simulink model "SimETC"  (R2025b)
settings: Solver=FixedStepAuto  StartTime=0.0  StopTime=50  FixedStep=Ts  RelTol=1e-3
values from neighbouring files (symbols this model uses):
  hiddenLayerSizeCtrl = 20    [Init.m]
  hiddenLayerSizeObsv = 5    [Init.m]
  n = 2    [Init.m]
  p = 1    [Init.m]
  Ts = 1e-3    (= 0.001)    [Init.m]
  u_max = 5    [Init.m]
  u_min = - 5    (= -5)    [Init.m]
  Vctrl0 = 0.1 * randn(hiddenLayerSizeCtrl, inputLayerSizeCtrl)    [Init.m]
  Vobsv0 = 0.1 * randn(hiddenLayerSizeObsv, inputLayerSizeObsv)    [Init.m]
  Wctrl0 = 0.1 * randn(outputLayerSizeCtrl, hiddenLayerSizeCtrl)    [Init.m]
  Wobsv0 = 0.1 * randn(outputLayerSizeObsv, hiddenLayerSizeObsv)    [Init.m]
  x0 = [0.5; 0]    [Init.m]
  x_hat0 = [0.9; 0]    [Init.m]
settings Model: Creator=Asus  LastModifiedBy=Asus

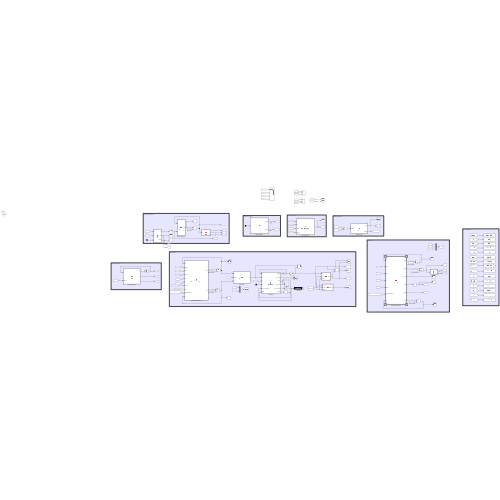
[thumbnail: Simulink's stored preview of the top-level diagram]
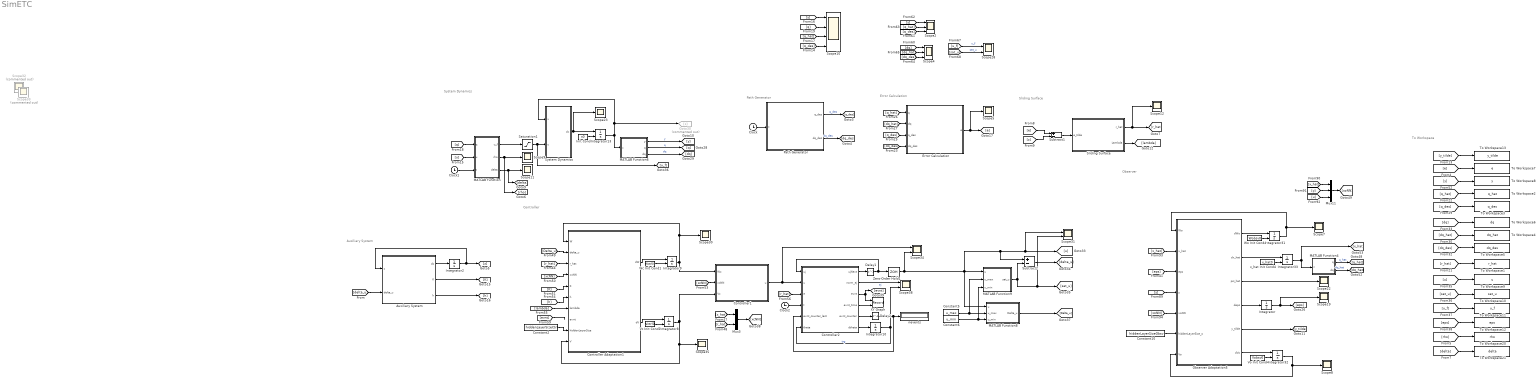
== system SimETC ==
  note: Path Generator
  note: Auxiliary System
  note: Sliding Surface
  note: Error Calculation
  note: Observer
  note: System Dynamics
  note: To Workspace
  note: Controller
  Auxiliary System : MATLAB Function  TreatAsAtomicUnit=on
  Clock : Clock
  Clock1 : Clock
  Clock2 : Clock
  Constant10 : Constant  Value=hiddenLayerSizeObsv
  Constant2 : Constant  Value=hiddenLayerSizeCtrl
  Constant5 : Constant  Value=u_max
  Constant6 : Constant  Value=u_min
  Controller Adaptation1 : MATLAB Function  TreatAsAtomicUnit=on
  Controller1 : MATLAB Function  TreatAsAtomicUnit=on
  Controller2 : MATLAB Function  TreatAsAtomicUnit=on
  Delay1 : Delay  DelayLength=1  InitialCondition=0  SampleTime=Ts
  Delay2 : Delay  DelayLength=1  InitialCondition=0  SampleTime=Ts
  Error Calculation : MATLAB Function  TreatAsAtomicUnit=on
  Goto30 : Goto  Commented=on  GotoTag=x
  Init Cond : Constant  Value=x0
  Integrator : Integrator  InitialCondition=5 * ones(p, 1)
  Integrator10 : Integrator  InitialCondition=1
  Integrator{13,31..33} (4 alike) : Integrator  InitialConditionSource=external  InitialCondition=[0.5; 0.5]
  Integrator2 : Integrator  InitialCondition=zeros(n, 1)
  Integrator8 : Integrator  InitialConditionSource=external
  Integrator9 : Integrator  InitialConditionSource=external
  MATLAB Function : MATLAB Function  TreatAsAtomicUnit=on
  MATLAB Function4 : MATLAB Function  TreatAsAtomicUnit=on
  MATLAB Function6 : MATLAB Function  TreatAsAtomicUnit=on
  MATLAB Function8 : MATLAB Function  TreatAsAtomicUnit=on
  MATLAB Function9 : MATLAB Function  TreatAsAtomicUnit=on
  Mux11 : Mux  Inputs=3
  Mux3 : Mux  Inputs=2
  Observer Adaptation5 : MATLAB Function  TreatAsAtomicUnit=on
  Path Generator : MATLAB Function  TreatAsAtomicUnit=on
  Saturation1 : Saturate  UpperLimit=u_max  LowerLimit=u_min
  Scope10 : Scope  NumInputPorts=4
      settings: ActiveDisplayYMinimum=-1.6367696892605232  ActiveDisplayYMaximum=1.5189809741527545  DataLoggingVariableName=ScopeData11
  Scope{5,7..9,11..12,19,22..23,30,35} (11 alike) : Scope
      Scope11 settings: ActiveDisplayYMinimum=-0.44130868539267287  ActiveDisplayYMaximum=0.66139690029774989  DataLoggingVariableName=ScopeData6
      Scope12 settings: ActiveDisplayYMinimum=-17.664742140770244  ActiveDisplayYMaximum=31.96274912675225  DataLoggingVariableName=ScopeData7
      Scope19 settings: ActiveDisplayYMinimum=1.4821345739344274  ActiveDisplayYMaximum=36.660788834590164  DataLoggingVariableName=ScopeData15
      Scope22 settings: ActiveDisplayYMinimum=-0.17253514431660325  ActiveDisplayYMaximum=0.24898535652907006  DataLoggingVariableName=ScopeData18
      Scope23 settings: ActiveDisplayYMinimum=-17.129349977314451  ActiveDisplayYMaximum=21.988712096819278  DataLoggingVariableName=ScopeData19
      Scope30 settings: ActiveDisplayYMinimum=-1.927386800082266  ActiveDisplayYMaximum=2.0755368522631517  DataLoggingVariableName=ScopeData29
      Scope35 settings: ActiveDisplayYMinimum=-1  ActiveDisplayYMaximum=1  DataLoggingVariableName=ScopeData34
      Scope5 settings: ActiveDisplayYMinimum=-0.81519678925710282  ActiveDisplayYMaximum=0.81279964325078913
      Scope7 settings: ActiveDisplayYMinimum=-0.11116662287651718  ActiveDisplayYMaximum=0.13560443561010163  DataLoggingVariableName=ScopeData9
      Scope8 settings: ActiveDisplayYMinimum=-0.37596192997099781  ActiveDisplayYMaximum=0.43937320774408428  DataLoggingVariableName=ScopeData10
      Scope9 settings: ActiveDisplayYMinimum=0.66977640233126912  ActiveDisplayYMaximum=1.0366915108520809  DataLoggingVariableName=ScopeData5
  Scope2 : Scope  NumInputPorts=3
      settings: ActiveDisplayYMinimum=-0.95485365659347476  ActiveDisplayYMaximum=1.1060948507326083
  Scope{28,31,34,38} (4 alike) : Scope  NumInputPorts=2
      Scope28 settings: ActiveDisplayYMinimum=-6.25  ActiveDisplayYMaximum=6.25  DataLoggingVariableName=ScopeData24
      Scope31 settings: ActiveDisplayYMinimum=-16.631670131101757  ActiveDisplayYMaximum=15.404984351853386  DataLoggingVariableName=ScopeData30
      Scope34 settings: ActiveDisplayYMinimum=-1.1199808946106344  ActiveDisplayYMaximum=-0.23536958662686125  DataLoggingVariableName=ScopeData33
      Scope38 settings: ActiveDisplayYMinimum=-0.40772759021012284  ActiveDisplayYMaximum=3.6695544974688574  DataLoggingVariableName=ScopeData37
  Scope32 : Scope  Commented=on
      settings: ActiveDisplayYMinimum=-0.12499999999999997  ActiveDisplayYMaximum=1.125  DataLoggingVariableName=ScopeData31
  Scope33 : Scope  Commented=on
      settings: ActiveDisplayYMinimum=-0.12499999999999997  ActiveDisplayYMaximum=1.125  DataLoggingVariableName=ScopeData32
  Scope4 : Scope  NumInputPorts=3
      settings: ActiveDisplayYMinimum=-2.1086647102859288  ActiveDisplayYMaximum=2.2459506500821029  DataLoggingVariableName=ScopeData8
  Sliding Surface : MATLAB Function  TreatAsAtomicUnit=on
  Subtract1 : Sum  Inputs=+-
  Subtract2 : Sum  Inputs=+-
  System Dynamics : MATLAB Function  TreatAsAtomicUnit=on
  To Workspace1 : ToWorkspace  VariableName=r_hat  SaveFormat=Structure  SampleTime=-1
      settings: Save2DSignal=2-D array (concatenate along first dimension)
  To Workspace10 : ToWorkspace  VariableName=sat_u  SaveFormat=Structure  SampleTime=-1
      settings: Save2DSignal=2-D array (concatenate along first dimension)
  To Workspace11 : ToWorkspace  VariableName=u_f  SaveFormat=Structure  SampleTime=-1
      settings: Save2DSignal=2-D array (concatenate along first dimension)
  To Workspace12 : ToWorkspace  VariableName=eps  SaveFormat=Structure  SampleTime=-1
      settings: Save2DSignal=2-D array (concatenate along first dimension)
  To Workspace13 : ToWorkspace  VariableName=y_tilde  SaveFormat=Structure  SampleTime=-1
      settings: Save2DSignal=2-D array (concatenate along first dimension)
  To Workspace2 : ToWorkspace  VariableName=q_hat  SaveFormat=Structure  SampleTime=-1
      settings: Save2DSignal=2-D array (concatenate along first dimension)
  To Workspace20 : ToWorkspace  VariableName=rho  SaveFormat=Structure  SampleTime=-1
      settings: Save2DSignal=2-D array (concatenate along first dimension)
  To Workspace21 : ToWorkspace  VariableName=delta  SaveFormat=Structure  SampleTime=-1
      settings: Save2DSignal=2-D array (concatenate along first dimension)
  To Workspace3 : ToWorkspace  VariableName=q_des  SaveFormat=Structure  SampleTime=-1
      settings: Save2DSignal=2-D array (concatenate along first dimension)
  To Workspace4 : ToWorkspace  VariableName=dq_hat  SaveFormat=Structure  SampleTime=-1
      settings: Save2DSignal=2-D array (concatenate along first dimension)
  To Workspace5 : ToWorkspace  VariableName=dq_des  SaveFormat=Structure  SampleTime=-1
      settings: Save2DSignal=2-D array (concatenate along first dimension)
  To Workspace6 : ToWorkspace  VariableName=dq  SaveFormat=Structure  SampleTime=-1
      settings: Save2DSignal=2-D array (concatenate along first dimension)
  To Workspace7 : ToWorkspace  VariableName=e  SaveFormat=Structure  SampleTime=-1
      settings: Save2DSignal=2-D array (concatenate along first dimension)
  To Workspace8 : ToWorkspace  VariableName=y  SaveFormat=Structure  SampleTime=-1
      settings: Save2DSignal=2-D array (concatenate along first dimension)
  To Workspace9 : ToWorkspace  VariableName=u  SaveFormat=Structure  SampleTime=-1
      settings: Save2DSignal=2-D array (concatenate along first dimension)
  Vc Init Cond1 : Constant  Value=Vctrl0
  Vo Init Cond4 : Constant  Value=Vobsv0
  Wc Init Cond1 : Constant  Value=Wctrl0
  Wo Init Cond4 : Constant  Value=Wobsv0
  XY Graph : Record  NumPorts=2.0  FileSettingsInternal="{\"entries\":[{\"content\":{\"excelSettings\":{\"content\":{},\"type\":\"Streamout.ExcelSettings\"},\"parquetSettings\":{\"content\":{},\"type\":\"Streamout.ParquetSettings\"}},\"type\":\"Streamout.FileSettingStorage\",\"uuid\":\"\"}],\"packageUris\":[\"http:\\/\\/schema.mathworks.com\\/mf0\\/streamout_blocks\\/R2020a\"],\"version\":\"1.0\"}"  FrameSettings=[0, 0]  Layout=[1 1]  SignalsInternal="{\"entries\":[{\"content\":{\"signals\":[{\"content\":{\"blockPath\":[],\"dimensions\":[1],\"domain\":\"\",\"lineColor\":\"#a2142f\",\"plots\":[ 1 ],\"port\":1,\"sid\":[\"\"],\"signalID\":1,\"signalName\":\"Controller2:3\"},\"type\":\"RecordBlkView.Signal\",\"uuid\":\"\"},{\"content\":{\"blockPath\":[],\"dimensions\":[1],\"domain\":\"\",\"lineColor\":\"#139fff\",\"plots\":[ 1 ],\"port\":2,\"sid\":[\"\"],\"signalID\":2,\"signalName\":\"Controller2:4\"},\"type\":\"RecordBlkView.Signal\",\"uuid\":\"\"}]},\"type\":\"RecordBlkView.InputSignals\",\"uuid\":\"\"}],\"packageUris\":[\"http:\\/\\/schema.mathworks.com\\/mf0\\/streamout_blocks\\/R2020a\"],\"version\":\"1.0\"}"  VisualizationBindings="{\"xyplotplugin\":{\"info\":[{\"series\":[{\"bindingParametersList\":[{\"parameter\":\"X-Axis\",\"signalID\":1,\"signalName\":\"Controller2:3\"},{\"parameter\":\"Y-Axis\",\"signalID\":2,\"signalName\":\"Controller2:4\"}],\"seriesID\":0}],\"subplotID\":1}]}}"  CompatibilityTag=XY
  Zero-Order Hold1 : ZeroOrderHold  SampleTime=Ts
  nevents : Display
  x_hat Init Cond4 : Constant  Value=x_hat0
  wires:
  Clock/1 -> Path Generator/1(t)
  Auxiliary System/1(dz) -> Integrator2/1
  Integrator2/1 -> [z], Auxiliary System/1(z)
  Sliding Surface/1(r_hat) -> Scope12/1, [r_hat]
  Path Generator/2(dq_des) -> [dq_des]  "dq_des"
  Path Generator/1(q_des) -> [q_des]  "q_des"
  Sliding Surface/2(Lambda) -> [lambda]
  Error Calculation/1(e) -> Scope5/1, [e]
  [q_des] -> Error Calculation/3(q_des)
  [dq_des] -> Error Calculation/4(dq_des)
  [delta_u] -> Auxiliary System/2(delta_u)
  [dq_hat] -> Error Calculation/2(dq)
  Observer Adaptation5/2(dx_hat) -> Integrator33/1
  Observer Adaptation5/6(dVo) -> Integrator32/1
  Mux11/1 -> [xoNN]
  MATLAB Function4/2(dq) -> [dq_hat]  "dq_hat"
  [xoNN] -> Observer Adaptation5/5(xoNN)
  Integrator32/1 -> Observer Adaptation5/7(Vo), Scope8/1
  MATLAB Function4/1(q) -> [q_hat]  "q_hat"
  [u] -> Mux11/3
  [y] -> Observer Adaptation5/4(y)
  Wo Init Cond4/1 -> Integrator31/2
  Constant10/1 -> Observer Adaptation5/6(hiddenLayerSize_o)
  [x_hat] -> Observer Adaptation5/2(x_hat)
  Integrator31/1 -> Scope7/1, Observer Adaptation5/1(Wo)
  x_hat Init Cond4/1 -> Integrator33/2
  [x_hat] -> Mux11/1
  Vo Init Cond4/1 -> Integrator32/2
  [y] -> Mux11/2
  [q_hat] -> Error Calculation/1(q)
  MATLAB Function6/2(q) -> [q]  "q"
  Integrator13/1 -> System Dynamics/1(x), Goto30/1, MATLAB Function6/1(x)
  System Dynamics/1(dx) -> Scope23/1, Integrator13/1
  MATLAB Function6/3(dq) -> [dq]  "dq"
  Init Cond/1 -> Integrator13/2
  Observer Adaptation5/1(dWo) -> Integrator31/1
  Integrator33/1 -> MATLAB Function4/1(x), [x_hat]
  Observer Adaptation5/4(deps) -> Integrator/1
  Integrator/1 -> Scope19/1, [eps]
  [eps] -> Observer Adaptation5/3(eps)
  Observer Adaptation5/3(psi_hat) -> Scope22/1
  [e] -> Subtract1/1
  Subtract1/1 -> Sliding Surface/1(e_tilde)
  [z] -> Subtract1/2
  [y] -> Scope2/1
  Saturation1/1 -> System Dynamics/2(u), [u_f]
  [u_f] -> Scope28/1  "u_f"
  [sat_u] -> Scope28/2  "sat_u"
  Clock1/1 -> MATLAB Function/3(t)
  [u] -> MATLAB Function/2(u)
  [q] -> MATLAB Function/1(q)
  MATLAB Function/2(rho) -> Scope9/1, [rho]
  MATLAB Function/3(delta) -> [delta], Scope11/1
  Auxiliary System/2(K) -> [K]
  Auxiliary System/3(h) -> [h]
  [q_hat] -> Scope2/2
  [q_des] -> Scope2/3
  [dq] -> Scope4/1
  [dq_hat] -> Scope4/2
  [dq_des] -> Scope4/3
  [dq_des] -> To Workspace5/1
  [q_des] -> To Workspace3/1
  [eps] -> To Workspace12/1
  [sat_u] -> To Workspace10/1
  [r_hat] -> To Workspace1/1
  [y] -> To Workspace8/1
  [u] -> To Workspace9/1
  [u_f] -> To Workspace11/1
  [dq] -> To Workspace6/1
  [dq_hat] -> To Workspace4/1
  [q_hat] -> To Workspace2/1
  [rho] -> To Workspace20/1
  [delta] -> To Workspace21/1
  [e] -> To Workspace7/1
  Observer Adaptation5/5(y_tilde) -> [y_tilde]
  [y_tilde] -> To Workspace13/1
  MATLAB Function6/1(y) -> [y]  "y"
  MATLAB Function/1(u_f) -> Saturation1/1
  [y] -> Scope10/1
  [q_hat] -> Scope10/3
  [q_des] -> Scope10/4
  [q] -> Scope10/2
  [K] -> Controller Adaptation1/5(K)
  [r_hat] -> Mux3/2
  [h] -> Controller Adaptation1/6(h)
  Constant2/1 -> Controller Adaptation1/9(hiddenLayerSize)
  Mux3/1 -> [xcNN]
  Integrator9/1 -> Controller1/1(Wc), Scope30/1, Controller Adaptation1/1(W)
  [Delta_u] -> Controller Adaptation1/2(delta_u)
  Integrator8/1 -> Controller1/3(Vc), Scope35/1, Controller Adaptation1/10(V)
  [lambda] -> Controller Adaptation1/7(lambda)
  [r_hat] -> Controller Adaptation1/3(r_hat)
  Wc Init Cond1/1 -> Integrator9/2
  [x_hat] -> Mux3/1
  [xcNN] -> Controller Adaptation1/4(xcNN)
  [xcNN] -> Controller1/2(xcNN)
  Controller2/1(ujNext) -> Delay1/1
  Delay1/1 -> Controller2/1(uj), Zero-Order Hold1/1
  MATLAB Function9/1(sat_u) -> Scope31/2, [sat_u], Subtract2/2
  Constant5/1 -> MATLAB Function9/2(u_max), MATLAB Function8/2(u_max)
  MATLAB Function8/1(Delta_u) -> [Delta_u]
  Constant6/1 -> MATLAB Function9/3(u_min), MATLAB Function8/3(u_min)
  Subtract2/1 -> [delta_u]
  Zero-Order Hold1/1 -> Scope34/2, MATLAB Function9/1(u), Scope31/1, [u], Subtract2/1, MATLAB Function8/1(u)
  Controller2/2(norm_ej) -> Scope38/1  "ej"
  [evnt] -> ?
  Vc Init Cond1/1 -> Integrator8/2
  Controller Adaptation1/2(dV) -> Integrator8/1
  Controller Adaptation1/1(dW) -> Integrator9/1
  Controller2/6(dtheta) -> Integrator10/1
  Clock2/1 -> Controller2/4(t)
  [r_hat] -> Controller2/3(e)
  Integrator10/1 -> Scope38/2, Controller2/6(theta)  "trg"
  Controller2/5(evnt_counter) -> Delay2/1
  Delay2/1 -> nevents/1, Controller2/5(evnt_counter_last)
  Controller2/3(evnt) -> XY Graph/1, [evnt]
  Controller2/4(evnt_time) -> XY Graph/2
  Controller1/1(u) -> Scope34/1, Controller2/2(u)

== matlab function SimETC/Sliding Surface ==
  data: e_tilde input; r_hat output; Lambda output
function [r_hat, Lambda] = SlidingSurface(e_tilde)

    Lambda = 30;

    r_hat = [Lambda, 1] * e_tilde;

end

== matlab function SimETC/Error Calculation ==
  data: e output; q input; dq input; q_des input; dq_des input
function e = ErrorCalculation(q, dq, q_des, dq_des)

    y_bar = [q(1); dq(1)];
    y_bar_des = [q_des(1); dq_des(1)];
    e = y_bar - y_bar_des;
    
end

== matlab function SimETC/MATLAB Function6 ==
  data: y output; x input; q output; dq output
function [y, q, dq] = fcn(x)

    q  = x(1);
    dq = x(2);
    % y  = exp(q)*sin(q) + q;
    y  = 0.3*q^3 - 0.5*q^2 + q;

end

== matlab function SimETC/System Dynamics ==
  data: x input; dx output; u input
function dx = Dynamics(x, u)

    A = [0, 1; 0, 0];
    B = [0; 1];

    % dynamics
    psi = (x(1) + x(2)) / (1 + (x(1) + x(2))^2) ...
    + (1 + x(2)^2) * x(1)^2 + x(1) * cos(x(1)) * sin(x(2)) ...
    + 0.5 * sin(x(2) * exp(-x(1)^2)) + log(3 + cos(x(1)) ...
    + sin(x(1)*x(2))^2) - log(1 + x(1)^2*x(2)^2) ...
    + (2 + cos(x(1)*x(2))) * u + 0.1*u^3 + sin(0.5*u) + tanh(u);
    dx  = A * x + B * psi;

    dx(1) = x(2) * (1 - 0.5 * cos(x(1)));

end

== matlab function SimETC/Controller Adaptation1 ==
  data: dW output; dV output; W input; delta_u input; r_hat input; xcNN input; K input; h input; lambda input; evnt input; hiddenLayerSize input; V input
function [dW, dV] = ControllerAdaptation(W, delta_u, r_hat, xcNN, K, h, lambda, evnt, hiddenLayerSize, V)
    
    Sigma = @(z) (-1 + 2 ./ (1 + exp(-2 * z)));
    Sigma_c  = Sigma(V * xcNN);

    l = 20;

    A = [0, 1; 0, 0];
    B = [0; 1];

    Ac = A - B * ([lambda', 1] * l + [0, lambda']);

    eta   = 10 * [0.1, 0.1];
    gamma = [0.0005, 0.0005];

    PI_c      = diag(Sigma_c.^2);
    PI_lambda = [lambda', 1];

    
    dW = eta(1) * (r_hat' * PI_lambda * (-Ac^(-1) * B + K^(-1) * h * diag(delta_u)))' * Sigma_c' - gamma(1) * norm(r_hat) * W';
    % dV = eta(2) * (r_hat' * PI_lambda * (-Ac^(-1) * B + K^(-1) * h * diag(delta_u)) * W' * (eye(hiddenLayerSize) - PI_c))' * xcNN' - gamma(2) * norm(r_hat) * V;

    dV = zeros(size(V));


end

== matlab function SimETC/MATLAB Function4 ==
  data: x input; q output; dq output
function [q, dq] = fcn(x)

    q  = x(1);
    dq = x(2);

end

== matlab function SimETC/Observer Adaptation5 ==
  data: dWo output; dx_hat output; psi_hat output; deps output; y_tilde output; dVo output; Wo input; x_hat input; eps input; y input; xoNN input; hiddenLayerSize_o input; Vo input
function [dWo, dx_hat, psi_hat, deps, y_tilde, dVo] = ObserverAdaptation(Wo, x_hat, eps, y, xoNN, hiddenLayerSize_o, Vo)

    Sigma = @(z) (-1 + 2 ./ (1 + exp(-2 * z)));
    Sigma_o = Sigma(Vo * xoNN);

    A = [0, 1; 0, 0];
    B = [0; 1];
    C = [1; 0];
    
    y_hat   = C' * x_hat;
    y_tilde = y - y_hat;

    alpha  = [1, 2];
    lambda = 0.01;
    kappa  = 50 ./ lambda;
    
    if abs(y_tilde) > lambda
        deps = kappa * y_tilde^2;
    else
        deps = 0;
    end
    
    rho = 2;
    Ho  = alpha(1, 2)*eps^rho;
    
    D = [alpha(1, 1)*eps; 0];
    
    Ao   = A  - D*C';
    Aocl = Ao - B*Ho*C';

    psi_hat = Wo' * Sigma_o;
    dx_hat  = Ao * x_hat + B * (psi_hat + Ho * y_tilde) + D * y;

    eta_o   = 2  * [10, 10];
    gamma_o = 10 * [0.01, 0.01];

    PI_o = diag(Sigma_o.^2);

    dWo = - eta_o(1) * (y_tilde' * C' * Aocl^(-1) * B)' * Sigma_o' - gamma_o(1) * norm(y_tilde) * Wo';
    % dVo = - eta_o(2) * (y_tilde' * C' * Aocl^(-1) * B * Wo' * (eye(hiddenLayerSize_o) - PI_o))' * xoNN' - gamma_o(2) * norm(y_tilde) * Vo;
    dVo = zeros(size(Vo));

end

== matlab function SimETC/Controller1 ==
  data: u output; Wc input; xcNN input; Vc input
function u = Controller(Wc, xcNN, Vc)

    Sigma = @(z) (-1 + 2 ./ (1 + exp(-2 * z)));
    u = - Wc' * Sigma(Vc * xcNN);
    
end

== matlab function SimETC/MATLAB Function8 ==
  data: u input; Delta_u output; u_max input; u_min input
function Delta_u = fcn(u, u_max, u_min)

    % if u > u_max
    %     Delta_u   = 1;
    % elseif u < u_min
    %     Delta_u   = 1;
    % else
    %     Delta_u   = 0;
    % end

    q       = 50;
    Delta_u = 1 - (1 + abs((u - (u_max+u_min)/2)/((u_max-u_min)/2))^q)^(-(q+1)/q);

end

== matlab function SimETC/MATLAB Function9 ==
  data: u input; sat_u output; u_max input; u_min input
function sat_u = fcn(u, u_max, u_min)

    q     = 50;
    sat_u = (u_max+u_min)/2 + (u - (u_max+u_min)/2) / (1 + abs((u - (u_max+u_min)/2)/((u_max-u_min)/2))^q)^(1/q);

end

== matlab function SimETC/Controller2 ==
  data: uj input; u input; e input; t input; ujNext output; norm_ej output; evnt output; evnt_time output; evnt_counter output; dtheta output; evnt_counter_last input; theta input
function [ujNext, norm_ej, evnt, evnt_time, evnt_counter, dtheta] = Controller(uj, u, e, t, evnt_counter_last, theta)

    ej = uj - u;
    norm_ej = norm(ej);

    lambda = 0.5;
    gamma  = 0.2;
    dtheta = - lambda * theta + gamma * norm(e);
    
    if norm(ej) > theta
        ujNext = u;
        evnt   = 1;
        evnt_counter = evnt_counter_last + 1;
        evnt_time = t;
    else
        ujNext = uj;
        evnt   = 0;
        evnt_counter = evnt_counter_last;
        evnt_time = 0;
    end
    
end

== matlab function SimETC/Auxiliary System ==
  data: z input; dz output; delta_u input; K output; h output
function [dz, K, h] = AuxiliarySystem(z, delta_u)
    
    K = 5  * diag([-1, -1]);
    h = 0.05 * [-1; -1];

    dz = K * z + h .* delta_u;
    
end

== matlab function SimETC/MATLAB Function ==
  data: q input; u input; u_f output; t input; rho output; delta output
function [u_f, rho, delta] = fcn(q, u, t)

    a     = 0.8;
    b     = 0.05;
    rho   = a + (1-a) * exp(-0.2 * t) + b * sin(10 * t) + b * cos(10 * t + sin(t) + pi/3) - b/2;
    % f = 0;
    % if t > 20 && t<30
    f = 0.3 * sin(t) - 0.2 * cos(2*(t))^2;
    % end
    delta = -(0.2 * cos(pi/3-tanh(q)^2) * sin(q) + f);
    u_f   = rho .* u + delta;

    u_f = u;

end

== matlab function SimETC/Path Generator ==
  data: t input; q_des output; dq_des output
function [q_des, dq_des] = PathGen(t)
    
    q_des   =   0.5 * cos(0.7 * t + pi/3) + 0.2 * sin(1.8 * t);
    dq_des  = - 0.5 * 0.7 * sin(0.7 * t + pi/3) + 0.2 * 1.8 * cos(1.8 * t);

    % q_des   = 0;
    % dq_des  = 0;
    
end
